simulink model "AGC30_PVcut_2021"  (R2021a)
settings: Solver=ode4  StartTime=stime  StopTime=etime  FixedStep=dtload  RelTol=1e-3
values from neighbouring files (symbols this model uses):
  AL_A = 0.3    [initset_lfc.m]
  AL_B = 0.3    [initset_lfc.m]
  DELTA_B = 0.067    [initset_otherarea.m]
  dtload = 0.1    [initset_dataload.m]
  F0 = 60    [initset_inertia.m]
  FFCS0_CC = (WF0_CC-WF_MIN_CC)./(1.0-WF_MIN_CC)    [init_thermals.m]
  FX_FB_ST_OA = Fx_fb_st_ty(:,TY_ST)    [initset_otherarea.m]
  FX_FB_WT = FX_FB_WT_ty(:,TY_WT)    [read_const_conhydros.m]
  FX_PTHD_ST_OA = Fx_pthd_st_ty(:,TY_ST)    [initset_otherarea.m]
  FY_FB_ST_OA = [1;1;0;0;-1;-1]*PLM_B    [initset_otherarea.m]
  FY_FB_WT = FY_FB_WT_ty(:,TY_WT)    [read_const_conhydros.m]
  FY_PTHD_ST_OA = [1;1;1;1]    [initset_otherarea.m]
  G_cost = [Cost(:,3) ... (first row only)    [initset_dataload.m]
  G_down_limit = max(G_down_limit, G_out_pre - G_speed*5)    [edc.m]    (also in initset_dataload.m = csvread('G_down_plan_limit.csv',0,1))
  G_G_ST_OA = G_g_st_ty(TY_ST)    [initset_otherarea.m]
  G_speed = u(220:249,1)    [edc.m]    (also in initset_dataload.m = G_speed(:,1))
  GF_CC = [1, 1, 1, 1, 1,            1, 1, 1, 1, 1]    [initset_thermals.m]
  GF_ST = [1, 1, 1, 1, 1, 1, 1,            1, 1, 1, 1,            1, 1, 1, 1, 1, 1]    [initset_thermals.m]
  GMW_WT = GMW_WT_ty(TY_WT)    [read_const_conhydros.m]
  IGV0_CC = WF0_CC    [init_thermals.m]
  inertia_input = [1 31.872 31.872 2 31.872 31.872 3 31.872 31.872 4 31.872 31.872 ... (259203 elements, 3x86401)]    [inertia_input.mat]    (also in initset_dataload.m = inertia_input')
  K1_CONV_WT = K1_CONV_WT_ty(TY_WT)    [read_const_conhydros.m]
  K2_SERV_WT = K2_SERV_WT_ty(TY_WT)    [read_const_conhydros.m]
  K_A = 0.1    [initset_lfc.m]
  K_B = 0.1    [initset_lfc.m]
  K_G_ST_OA = K_g_st_ty(TY_ST)    [initset_otherarea.m]
  K_L = 2.0    (= 2)    [initset_inertia.m]
  K_PREF_ST_OA = K_pref_st_ty(TY_ST)    [initset_otherarea.m]
  K_SD_WT = K_SD_WT_ty(TY_WT)    [read_const_conhydros.m]
  K_SEQ_WT = K_SEQ_WT_ty(TY_WT)    [read_const_conhydros.m]
  KD_PID_WT = KD_PID_WT_ty(TY_WT)    [read_const_conhydros.m]
  KGT_CC = FGT_CC./((TFR_CC-TER_CC)-(TDR_CC-TIR_CC))    [init_thermals.m]
  KI_PID_WT = KI_PID_WT_ty(TY_WT)    [read_const_conhydros.m]
  KP_A = 1.0    (= 1)    [initset_lfc.m]
  KP_B = 1.0    (= 1)    [initset_lfc.m]
  KP_PID_WT = KP_PID_WT_ty(TY_WT)    [read_const_conhydros.m]
  KST_CC = (1.0-FGT_CC)./TER_CC    [init_thermals.m]
  L_MWD_WT = L_MWD_WT_ty(TY_WT)    [read_const_conhydros.m]
  LFC_cycle = 5.0    (= 5)    [initset_lfc.m]
  load_input = load_input(:,stime+1:etime+1)    [initset_dataload.m]
  MVABase = 1000    [initset_inertia.m]
  MW0_ST = zeros(1,17)    [init_thermals.m]
  MW0_WT = zeros(1,2)    [init_conhydros.m]
  P_G_CONV_WT = P_G_CONV_WT_ty(TY_WT)    [read_const_conhydros.m]
  PG_INIT_CC = PMWD_SCHEDULE(1,19:28)'    [init_thermals.m]
  PLM_B = 0.03    [initset_otherarea.m]
  PMAX_B = 360.0    (= 360)    [initset_lfc.m]
  PMIN_B = -360.0    (= -360)    [initset_lfc.m]
  PMST0_CC = zeros(1, 10)    [init_thermals.m]
  PMWD_EDC0 = zeros(1,30)    [initset_edc.m]
  PMWD_SCHEDULE = u(3:32,1)    [edc.m]    (also in initset_edc.m = g_out_input')
  PRT_CC = PRC_CC.*(1-EP_CC)    [init_thermals.m]
  PTH0_ST = zeros(1,17)    [init_thermals.m]
  R_LL_ST_OA = R_ll_st_ty(TY_ST)    [initset_otherarea.m]
  RA_A = G_speed'    [initset_lfc.m]
  RA_B = 96.0    (= 96)    [initset_lfc.m]
  T1_B_ST_OA = T1_b_st_ty(TY_ST)    [initset_otherarea.m]
  T1_CONV_WT = T1_CONV_WT_ty(TY_WT)    [read_const_conhydros.m]
  T1_G_ST_OA = T1_g_st_ty(TY_ST)    [initset_otherarea.m]
  T2_B_ST_OA = T2_b_st_ty(TY_ST)    [initset_otherarea.m]
  T2_G_ST_OA = T2_g_st_ty(TY_ST)    [initset_otherarea.m]
  T2_SERV_WT = T2_SERV_WT_ty(TY_WT)    [read_const_conhydros.m]
  T3_B_ST_OA = T3_b_st_ty(TY_ST)    [initset_otherarea.m]
  T3_SERV_WT = T3_SERV_WT_ty(TY_WT)    [read_const_conhydros.m]
  T4_G_ST_OA = T4_g_st_ty(TY_ST)    [initset_otherarea.m]
  T5_G_ST_OA = T5_g_st_ty(TY_ST)    [initset_otherarea.m]
  T_0 = 2.5    [initset_trfpP.m]
  T_LL_ST_OA = T_ll_st_ty(TY_ST)    [initset_otherarea.m]
  T_PREF_ST_OA = T_pref_st_ty(TY_ST)    [initset_otherarea.m]
  TD_PID_WT = TD_PID_WT_ty(TY_WT)    [read_const_conhydros.m]
  TDR_CC = TIR_CC.*(1+(PRC_CC.^((RC_CC-1)./RC_CC)-1)./HC_CC)    [init_thermals.m]
  TE0_CC = zeros(1, 10)    [init_thermals.m]
  TER_CC = TFR_CC.*(1-(1-1./PRT_CC.^((RT_CC-1)./RT_CC)).*HT_CC)    [init_thermals.m]
  Tieline_Base = [1 0 2 0 3 0 4 0 5 0 6 0 ... (172802 elements, 2x86401)]    [Tieline_Base.mat]    (also in initset_dataload.m = Tieline_Base')
  TW_WAY_WT = TW_WAY_WT_ty(TY_WT)    [read_const_conhydros.m]
  U_MWD_WT = U_MWD_WT_ty(TY_WT)    [read_const_conhydros.m]
  WF0_CC = 1.0*ones(1, 10)    [init_thermals.m]
  WF_MIN_CC = L_IGV_CC./(TFR_CC-TDR_CC).*((Td_min_cc-TIR_CC)     ./((1-1./(PRT_CC.*L_IGV_CC).^((RT_CC-1)./RT_CC)).*HT_CC)-Td_min_cc)    [init_thermals.m]
  XAR_A = 10.0    (= 10)    [initset_lfc.m]
  XAR_B = 10.0    (= 10)    [initset_lfc.m]
  XF_A = 0.00    (= 0)    [initset_lfc.m]
  XF_B = 0.00    (= 0)    [initset_lfc.m]
undefined symbols (not defined in the file or in its folder): DELTA_CC, DELTA_ST, DiscIntNeverNeededParam, FGT_CC, FX_FB_CC, FX_FB_ST, FX_N_GN_VA, FX_N_PM_VA, FX_PTHD_ST, FX_T_PM_VA, FX_TE1_CC, FX_TE2_CC, FX_Y_GN_VA, FX_Y_PM_VA, FY_FB_CC, FY_FB_ST, FY_N_GN_VA, FY_N_PM_VA, FY_PTHD_ST, FY_T_PM_VA, FY_TE1_CC, FY_TE2_CC, FY_Y_GN_VA, FY_Y_PM_VA, G_G_ST, GMW_CC, GMW_ST, GMW_VA, HC_CC, HT_CC, K1_CONV_VA, K2_SERV_VA, K_G_ST, K_IGV_CC, K_MW_GV_VA, K_PREF_ST, K_SD_VA, K_TE_CC, KD_PID_VA, KD_SG_GN_VA, KD_SG_PM_VA, KI_PID_VA, KI_SG_GN_VA, KI_SG_PM_VA, KP_PID_VA, KP_SG_GN_VA, KP_SG_PM_VA, L_FUEL_CC, L_G_ST, L_IGV_CC, L_LL_ST, L_MWD_CC, L_MWD_GN_VA, L_MWD_PM_VA, L_MWD_ST, L_PREF_CC, L_PREF_ST, M_VA, MW0_ST_OA, N_GN_INIT_VA ... (+56)
libraries: simulink_extras x87, simulink x43, eeGeneralControl x2, pid_lib x1
(part 2 of 4)

== system AGC30_PVcut_2021/他エリア発電プラント/他エリアモデル ==
  EDC指令値(MW) : Inport
  LFC指令値(MW) : Inport  Port=2
  周波数偏差(Hz) : Inport  Port=3
  Add2 : Sum
  Add3 : Sum
  CVサーボ時定数 : Gain  Gain=1/T2_G_ST_OA(1)
  GF・LL幅 : Constant  Value=PLM_B
  Hz->pu : Gain  Gain=1/F0
  MW->pu : Product  Inputs=/*
  MWD' : Sum
  MWD(MW) : Sum
  MinMax : MinMax  Inputs=2
  Mux1 : Mux  Inputs=3
  Scope : Scope
  Subtract : Sum  Inputs=+-
  Subtract1 : Sum  Inputs=+-
  Subtract2 : Sum  Inputs=+-
  pu->MW : Product  RndMeth=Zero
  スピードリレー : TransferFcn  Numerator=[G_G_ST_OA(1) 1]  Denominator=[T1_G_ST_OA(1) 1]
  タービン出力 : Sum
  ボイラ特性 : simulink_extras/Additional Linear/Transfer Fcn (with initial outputs)  N=[1]  D=[T2_B_ST_OA(1) 1]  Y0=0  U0=0
  ボイラ発生蒸気 : simulink_extras/Additional Linear/Transfer Fcn (with initial outputs)  N=[1]  D=[T1_B_ST_OA(1) 1]  Y0=MW0_ST_OA(1)  U0=MW0_ST_OA(1)
  中低圧タービン・再熱器 : simulink_extras/Additional Linear/Transfer Fcn (with initial outputs)  N=[1]  D=[T5_G_ST_OA(1) 1]  Y0=MW0_ST_OA(1)  U0=MW0_ST_OA(1)
  中低圧タービン分担比 : Gain  Gain=1.0-K_G_ST_OA(1)
  主蒸気圧力 : Sum
  主蒸気圧力 偏差 : Sum  Inputs=+-
  主蒸気圧力設定 : Lookup  InputValues=FX_PTHD_ST_OA(:,1)  Table=FY_PTHD_ST_OA(:,1)  LookUpMeth=Interpolation-Use End Values
  主蒸気流量 : Product  RndMeth=Zero
  他エリア出力 : ToWorkspace  VariableName=OtherArea_Out  SampleTime=-1
      settings: Save2DSignal=2-D array (concatenate along first dimension)
  出力偏差 : Sum  Inputs=-++
  出力制御積分 : Integrator  InitialCondition=1.0  UpperSaturationLimit=Inf  LowerSaturationLimit=0
  周波数バイアス : Lookup  InputValues=FX_FB_ST_OA(:,1)/F0  Table=FY_FB_ST_OA(:,1)  LookUpMeth=Interpolation-Use End Values
  圧力制御 : simulink_extras/Additional Linear/Transfer Fcn (with initial outputs)  N=[1]  D=[T3_B_ST_OA(1) 1]  Y0=0  U0=0
  比例ゲイン : Gain  Gain=K_PREF_ST_OA(1)
  積分時定数 : Gain  Gain=1/T_PREF_ST_OA(1)
  蒸気加減弁開度 : Integrator  InitialCondition=1.0  UpperSaturationLimit=Inf  LowerSaturationLimit=0
  追従回路 : Subsystem
  速度調定率 : Gain  Gain=1.0/DELTA_B
  高圧タービン : simulink_extras/Additional Linear/Transfer Fcn (with initial outputs)  N=[1]  D=[T4_G_ST_OA(1) 1]  Y0=MW0_ST_OA(1)  U0=MW0_ST_OA(1)
  高圧タービン分担比 : Gain  Gain=K_G_ST_OA(1)
  タービン出力(MW) : Outport  VectorParamsAs1DForOutWhenUnconnected=off
  wires:
  MWD(MW)/1 -> MW->pu/2
  周波数偏差(Hz)/1 -> Hz->pu/1
  MWD'/1 -> ボイラ発生蒸気/1, 出力偏差/2
  ボイラ発生蒸気/1 -> Subtract/1, 主蒸気圧力設定/1
  出力偏差/1 -> 比例ゲイン/1, 積分時定数/1
  比例ゲイン/1 -> Add3/1
  主蒸気圧力 偏差/1 -> 主蒸気圧力/1, 出力偏差/3
  主蒸気圧力設定/1 -> 主蒸気圧力/2
  主蒸気流量/1 -> Subtract/2, 高圧タービン/1
  積分時定数/1 -> 出力制御積分/1
  出力制御積分/1 -> Add3/2
  速度調定率/1 -> スピードリレー/1
  Subtract1/1 -> MinMax/2
  主蒸気圧力/1 -> 主蒸気流量/1
  スピードリレー/1 -> Subtract1/2
  MinMax/1 -> Subtract2/1, Add2/2
  Subtract2/1 -> CVサーボ時定数/1
  CVサーボ時定数/1 -> 蒸気加減弁開度/1
  蒸気加減弁開度/1 -> 主蒸気流量/2, Subtract2/2
  高圧タービン/1 -> 中低圧タービン・再熱器/1, 高圧タービン分担比/1
  中低圧タービン・再熱器/1 -> 中低圧タービン分担比/1
  高圧タービン分担比/1 -> タービン出力/2
  中低圧タービン分担比/1 -> タービン出力/1
  タービン出力/1 -> pu->MW/1, 出力偏差/1
  GF・LL幅/1 -> Add2/1
  Add2/1 -> 追従回路/1(In)
  ボイラ特性/1 -> 主蒸気圧力 偏差/1
  圧力制御/1 -> 主蒸気圧力 偏差/2
  Subtract/1 -> ボイラ特性/1, 圧力制御/1
  Add3/1 -> Subtract1/1
  Hz->pu/1 -> 速度調定率/1, 周波数バイアス/1
  EDC指令値(MW)/1 -> Mux1/1, MW->pu/1, MWD(MW)/1, pu->MW/2
  LFC指令値(MW)/1 -> Mux1/2, MWD(MW)/2
  追従回路/1(Out) -> MinMax/1
  周波数バイアス/1 -> MWD'/1
  Mux1/1 -> 他エリア出力/1
  MW->pu/1 -> MWD'/2
  pu->MW/1 -> Scope/1, Mux1/3, タービン出力(MW)/1

== system AGC30_PVcut_2021/可変速揚水発電機/可変速揚水 ==
  note: EDCとLFC指令の入力方法を変更
  EDC指令値 (MW) : Inport
  LFC指令値 (MW) : Inport  Port=2
  周波数偏差 (Hz) : Inport  Port=3
  "  ±1  " : Saturate  UpperLimit=1  LowerLimit=-1
  " ±1 " : Integrator  LimitOutput=on  UpperSaturationLimit=1  LowerSaturationLimit=-1
  Abs : Abs
  Constant : Constant  Value=0
  EDC_Wt3 : Selector  InputPortWidth=AGCNum_E  IndexOptions=Index vector (dialog)  Indices=[30]  OutputSizes=1
  "Hz -> PU" : Gain  Gain=1/F0
  If : If  IfExpression=u1 >= 0
  LFC_Wt3 : Selector  InputPortWidth=AGCNum_L  IndexOptions=Index vector (dialog)  Indices=[30]  OutputSizes=1
  "MW -> PU" : Gain  Gain=1/GMW_VA(1)
  "PU -> MW" : Gain  Gain=GMW_VA(1)
  "SW " : Switch  Criteria=u2 > Threshold
  Scope{,1,3..6} (6 alike) : Scope
  Sum : Sum  Inputs=+++
  Sum2 : Sum  Inputs=|+-
  Sum3 : Sum  Inputs=|+-
  Sum4 : Sum
  Sum6 : Sum  Inputs=+|+
  ±1 : Saturate  UpperLimit=1  LowerLimit=-1
  微分 （リセットフィルタ） : TransferFcn  Numerator="[TD_PID_VA(1)  0]"  Denominator="[TD_PID_VA(1)  1]"
  微分ゲイン : Gain  Gain=KD_PID_VA(1)
  揚水運転 : Subsystem  TreatAsAtomicUnit=on
  比例ゲイン : Gain  Gain=KP_PID_VA(1)
  発電運転 : Subsystem  TreatAsAtomicUnit=on
  積分ゲイン : Gain  Gain=KI_PID_VA(1)
  速度調停率 : Gain  Gain=K_SD_VA(1)
  連続出力切替 : Subsystem
  運転モード : simulink/Logic and Bit Operations/Compare To Constant  relop=>=  const=GMW_VA(1)*L_MWD_GN_VA(1)  OutDataTypeStr=boolean
  発電機出力・揚水入力 (MW) : Outport  VectorParamsAs1DForOutWhenUnconnected=off
  wires:
  "MW -> PU"/1 -> Scope4/1, Sum2/1, 連続出力切替/3(MWD)
  EDC_Wt3/1 -> Abs/1, Scope6/1, 運転モード/1, Sum4/1
  Sum4/1 -> "MW -> PU"/1
  比例ゲイン/1 -> ±1/1
  Sum3/1 -> 微分ゲイン/1, 積分ゲイン/1, 比例ゲイン/1
  ±1/1 -> Sum/1
  " ±1 "/1 -> Sum/2
  積分ゲイン/1 -> " ±1 "/1
  EDC指令値 (MW)/1 -> EDC_Wt3/1
  "PU -> MW"/1 -> 発電機出力・揚水入力 (MW)/1
  連続出力切替/1(出力) -> "PU -> MW"/1
  揚水運転/1(Out2) -> Sum6/2, Scope1/1
  Sum6/1 -> Scope3/1, 連続出力切替/1(モデル)
  LFC_Wt3/1 -> Sum4/2
  LFC指令値 (MW)/1 -> LFC_Wt3/1
  微分ゲイン/1 -> 微分 （リセットフィルタ）/1
  運転モード/1 -> Scope5/1, 連続出力切替/2(運転モード)
  "  ±1  "/1 -> Sum/3
  速度調停率/1 -> Sum3/2
  "Hz -> PU"/1 -> Sum3/1
  周波数偏差 (Hz)/1 -> "Hz -> PU"/1
  微分 （リセットフィルタ）/1 -> "  ±1  "/1
  Sum/1 -> Sum2/2, 速度調停率/1
  Sum2/1 -> "SW "/1  "有効電力指令"
  Constant/1 -> "SW "/3
  Abs/1 -> "SW "/2
  If/1 -> 発電運転/Action
  If/2 -> 揚水運転/Action
  "SW "/1 -> 発電運転/1(In1), 揚水運転/1(In1), If/1
  発電運転/1(Out1) -> Scope/1, Sum6/1

== system AGC30_PVcut_2021/定速揚水発電プラント/Water1 ==
  note: IMAICHI P/S DYNAMIC BLOCK (imaichtd)
  EDC指令値(MW) : Inport
  LFC指令値(MW)1 : Inport  Port=2
  周波数偏差(Hz)1 : Inport  Port=3
  (1-TWs)/(1+0.5TWs) : simulink_extras/Additional Linear/Transfer Fcn (with initial outputs)  N=[-TW_WAY_WT(1) 1]  D=[TW_WAY_WT(1)/2 1]  Y0=MW0_WT(1)  U0=MW0_WT(1)
  Add : Sum
  Hz->pu : Gain  Gain=1/F0
  K1/(1+T1s)1 : simulink_extras/Additional Linear/Transfer Fcn (with initial outputs)  N=[K1_CONV_WT(1)]  D=[T1_CONV_WT(1) 1]  Y0=MW0_WT(1)/P_G_CONV_WT(1)  U0=MW0_WT(1)/P_G_CONV_WT(1)
  K2/(1+T2s+T3s^2)1 : simulink_extras/Additional Linear/Transfer Fcn (with initial outputs)  N=[K2_SERV_WT(1)]  D=[T3_SERV_WT(1) T2_SERV_WT(1) 1]  Y0=MW0_WT(1)/P_G_CONV_WT(1)  U0=MW0_WT(1)/P_G_CONV_WT(1)
  Kc/Tc (1/90) : Gain  Gain=K_SEQ_WT(1)  SaturateOnIntegerOverflow=on  OutDataTypeStr=Inherit: Same as input  ParamDataTypeStr=Inherit: Same as input
  Kd : Gain  Gain=KD_PID_WT(1)  SaturateOnIntegerOverflow=on  OutDataTypeStr=Inherit: Same as input  ParamDataTypeStr=Inherit: Same as input
  Ki : Gain  Gain=KI_PID_WT(1)  SaturateOnIntegerOverflow=on  OutDataTypeStr=Inherit: Same as input  ParamDataTypeStr=Inherit: Same as input
  Kp : Gain  Gain=KP_PID_WT(1)  SaturateOnIntegerOverflow=on  OutDataTypeStr=Inherit: Same as input  ParamDataTypeStr=Inherit: Same as input
  Ksd : Gain  Gain=K_SD_WT(1)  SaturateOnIntegerOverflow=on  OutDataTypeStr=Inherit: Same as input  ParamDataTypeStr=Inherit: Same as input
  MW->pu : Gain  Gain=1/GMW_WT(1)
  MWD(MW) : Sum
  Scope : Scope
  Scope1 : Scope
  Scope2 : Scope
  Scope4 : Scope  Commented=on
  Scope5 : Scope  Commented=on
  Sum12 : Sum  Inputs=-+  InputSameDT=on  SaturateOnIntegerOverflow=on  OutDataTypeStr=Inherit: Same as first input
  Sum17 : Sum  Inputs=-+  InputSameDT=on  SaturateOnIntegerOverflow=on  OutDataTypeStr=Inherit: Same as first input
  Sum18 : Sum  Inputs=-+  InputSameDT=on  SaturateOnIntegerOverflow=on  OutDataTypeStr=Inherit: Same as first input
  Sum19 : Sum  Inputs=+++  InputSameDT=on  SaturateOnIntegerOverflow=on  OutDataTypeStr=Inherit: Same as first input
  Tds/(1+Tds) : TransferFcn  Numerator=[TD_PID_WT(1) 0]  Denominator=[TD_PID_WT(1) 1]
  To Workspace : ToWorkspace  Commented=on  VariableName=PG1  SampleTime=-1
  To Workspace1 : ToWorkspace  Commented=on  VariableName=ELD  SampleTime=-1
  U=1  L=0 : Saturate  UpperLimit=1.  LowerLimit=0
  U=1 L=0 : Saturate  UpperLimit=1.  LowerLimit=0
  U=1.2L=1 : Subsystem  mask(Limited Integrator.){lower_limit=0, upper_limit=1.2, X0=MW0_WT(1)/P_G_CONV_WT(1)}
      mask prompts: lower_limit "Lower bound:"; upper_limit "Upper bound:"; X0 "Initial condition:"
      mask help: Limited Integrator
      mask Help: Implements a limited integrator with \nan expression of the form:\n\nif(x<=lb and u<0) or (x>=ub and u>0)\n   xdot=0\nelse\n   xdot=u
      mask Display: plot(-1,-0.2,3.5,1.2,[0.05,1,2,2.9],[0,0,1,1]);disp(' 1/s    ')
  U=1L=0 : Subsystem  mask(Limited Integrator.){lower_limit=0, upper_limit=1., X0=MW0_WT(1)/P_G_CONV_WT(1)}
      mask prompts: lower_limit "Lower bound:"; upper_limit "Upper bound:"; X0 "Initial condition:"
      mask help: Limited Integrator
      mask Help: Implements a limited integrator with \nan expression of the form:\n\nif(x<=lb and u<0) or (x>=ub and u>0)\n   xdot=0\nelse\n   xdot=u
      mask Display: plot(-1,-0.2,3.5,1.2,[0.05,1,2,2.9],[0,0,1,1]);disp(' 1/s    ')
  pu->MW : Gain  Gain=GMW_WT(1)  SaturateOnIntegerOverflow=on  OutDataTypeStr=Inherit: Same as input  ParamDataTypeStr=Inherit: Same as input
  puMW/puGV : Gain  Gain=P_G_CONV_WT(1)  SaturateOnIntegerOverflow=on  OutDataTypeStr=Inherit: Same as input  ParamDataTypeStr=Inherit: Same as input
  ±0.05 : Saturate  UpperLimit=0.05  LowerLimit=-0.05
  ±1 : Saturate  UpperLimit=1.  LowerLimit=-1.
  "±1 " : Saturate  UpperLimit=1.  LowerLimit=-1.
  出力上下限 : Saturate  UpperLimit=U_MWD_WT(1)  LowerLimit=L_MWD_WT(1)
  周波数バイアス : Lookup  InputValues=FX_FB_WT(:,1)/F0  Table=FY_FB_WT(:,1)  LookUpMeth=Interpolation-Use End Values
  連続出力切替 : Subsystem
  運転モード : simulink/Logic and Bit Operations/Compare To Constant  relop=>=  const=L_MWD_WT(1)*GMW_WT(1)  OutDataTypeStr=boolean
  タービン出力(MW) : Outport  VectorParamsAs1DForOutWhenUnconnected=off
  wires:
  ±0.05/1 -> Kc/Tc (1/90)/1
  Kc/Tc (1/90)/1 -> U=1.2L=1/1(Inport)
  U=1 L=0/1 -> Sum17/1, K2/(1+T2s+T3s^2)1/1
  Sum19/1 -> K1/(1+T1s)1/1
  U=1L=0/1(Outport) -> Sum19/2
  ±1/1 -> Sum19/1
  "±1 "/1 -> Sum19/3
  Tds/(1+Tds)/1 -> "±1 "/1
  Kd/1 -> Tds/(1+Tds)/1
  Kp/1 -> ±1/1
  Ki/1 -> U=1L=0/1(Inport)
  Sum17/1 -> Ksd/1
  Sum12/1 -> ±0.05/1
  Sum18/1 -> Ki/1, Kd/1, Kp/1
  U=1.2L=1/1(Outport) -> Sum17/2
  Ksd/1 -> Sum18/2
  K1/(1+T1s)1/1 -> U=1 L=0/1
  K2/(1+T2s+T3s^2)1/1 -> U=1  L=0/1
  出力上下限/1 -> Sum12/2
  EDC指令値(MW)/1 -> MWD(MW)/1, 運転モード/1, Scope2/1, To Workspace1/1
  LFC指令値(MW)1/1 -> MWD(MW)/2
  MWD(MW)/1 -> MW->pu/1
  周波数偏差(Hz)1/1 -> Hz->pu/1
  Hz->pu/1 -> 周波数バイアス/1, Sum18/1, Scope/1
  周波数バイアス/1 -> Add/2, Scope4/1
  MW->pu/1 -> Add/1, Scope1/1, 連続出力切替/3(MWD)
  Add/1 -> 出力上下限/1, Scope5/1
  U=1  L=0/1 -> puMW/puGV/1
  puMW/puGV/1 -> (1-TWs)/(1+0.5TWs)/1
  (1-TWs)/(1+0.5TWs)/1 -> Sum12/1, 連続出力切替/1(モデル)
  運転モード/1 -> 連続出力切替/2(運転モード)
  pu->MW/1 -> タービン出力(MW)/1, To Workspace/1
  連続出力切替/1(出力) -> pu->MW/1

== system AGC30_PVcut_2021/定速揚水発電プラント/Water2 ==
  EDC指令値(MW) : Inport
  LFC指令値(MW)1 : Inport  Port=2
  周波数偏差(Hz)1 : Inport  Port=3
  (1-TWs)/(1+0.5TWs) : simulink_extras/Additional Linear/Transfer Fcn (with initial outputs)  N=[-TW_WAY_WT(2) 1]  D=[TW_WAY_WT(2)/2 1]  Y0=MW0_WT(2)  U0=MW0_WT(2)
  Add : Sum
  Hz->pu : Gain  Gain=1/F0
  K1/(1+T1s)1 : simulink_extras/Additional Linear/Transfer Fcn (with initial outputs)  N=[K1_CONV_WT(2)]  D=[T1_CONV_WT(2) 1]  Y0=MW0_WT(2)/P_G_CONV_WT(2)  U0=MW0_WT(2)/P_G_CONV_WT(2)
  K2/(1+T2s+T3s^2)1 : simulink_extras/Additional Linear/Transfer Fcn (with initial outputs)  N=[K2_SERV_WT(2)]  D=[T3_SERV_WT(2) T2_SERV_WT(2) 1]  Y0=MW0_WT(2)/P_G_CONV_WT(2)  U0=MW0_WT(2)/P_G_CONV_WT(2)
  Kc/Tc (1/90) : Gain  Gain=K_SEQ_WT(2)  SaturateOnIntegerOverflow=on  OutDataTypeStr=Inherit: Same as input  ParamDataTypeStr=Inherit: Same as input
  Kd : Gain  Gain=KD_PID_WT(2)  SaturateOnIntegerOverflow=on  OutDataTypeStr=Inherit: Same as input  ParamDataTypeStr=Inherit: Same as input
  Ki : Gain  Gain=KI_PID_WT(2)  SaturateOnIntegerOverflow=on  OutDataTypeStr=Inherit: Same as input  ParamDataTypeStr=Inherit: Same as input
  Kp : Gain  Gain=KP_PID_WT(2)  SaturateOnIntegerOverflow=on  OutDataTypeStr=Inherit: Same as input  ParamDataTypeStr=Inherit: Same as input
  Ksd : Gain  Gain=K_SD_WT(2)  SaturateOnIntegerOverflow=on  OutDataTypeStr=Inherit: Same as input  ParamDataTypeStr=Inherit: Same as input
  MW->pu : Gain  Gain=1/GMW_WT(2)
  MWD(MW) : Sum
  Scope : Scope
  Scope1 : Scope  Commented=on
  Scope4 : Scope
  Scope5 : Scope  Commented=on
  Sum12 : Sum  Inputs=-+  InputSameDT=on  SaturateOnIntegerOverflow=on  OutDataTypeStr=Inherit: Same as first input
  Sum17 : Sum  Inputs=-+  InputSameDT=on  SaturateOnIntegerOverflow=on  OutDataTypeStr=Inherit: Same as first input
  Sum18 : Sum  Inputs=-+  InputSameDT=on  SaturateOnIntegerOverflow=on  OutDataTypeStr=Inherit: Same as first input
  Sum19 : Sum  Inputs=+++  InputSameDT=on  SaturateOnIntegerOverflow=on  OutDataTypeStr=Inherit: Same as first input
  Tds/(1+Tds) : TransferFcn  Numerator=[TD_PID_WT(2) 0]  Denominator=[TD_PID_WT(2) 1]
  U=1  L=0 : Saturate  UpperLimit=1.  LowerLimit=0
  U=1 L=0 : Saturate  UpperLimit=1.  LowerLimit=0
  U=1.2L=1 : Subsystem  mask(Limited Integrator.){lower_limit=0, upper_limit=1.2, X0=MW0_WT(2)/P_G_CONV_WT(2)}
      mask prompts: lower_limit "Lower bound:"; upper_limit "Upper bound:"; X0 "Initial condition:"
      mask help: Limited Integrator
      mask Help: Implements a limited integrator with \nan expression of the form:\n\nif(x<=lb and u<0) or (x>=ub and u>0)\n   xdot=0\nelse\n   xdot=u
      mask Display: plot(-1,-0.2,3.5,1.2,[0.05,1,2,2.9],[0,0,1,1]);disp(' 1/s    ')
  U=1L=0 : Subsystem  mask(Limited Integrator.){lower_limit=0, upper_limit=1., X0=MW0_WT(1)/P_G_CONV_WT(1)}
      mask prompts: lower_limit "Lower bound:"; upper_limit "Upper bound:"; X0 "Initial condition:"
      mask help: Limited Integrator
      mask Help: Implements a limited integrator with \nan expression of the form:\n\nif(x<=lb and u<0) or (x>=ub and u>0)\n   xdot=0\nelse\n   xdot=u
      mask Display: plot(-1,-0.2,3.5,1.2,[0.05,1,2,2.9],[0,0,1,1]);disp(' 1/s    ')
  pu->MW : Gain  Gain=GMW_WT(2)  SaturateOnIntegerOverflow=on  OutDataTypeStr=Inherit: Same as input  ParamDataTypeStr=Inherit: Same as input
  puMW/puGV : Gain  Gain=P_G_CONV_WT(2)  SaturateOnIntegerOverflow=on  OutDataTypeStr=Inherit: Same as input  ParamDataTypeStr=Inherit: Same as input
  ±0.05 : Saturate  UpperLimit=0.05  LowerLimit=-0.05
  ±1 : Saturate  UpperLimit=1.  LowerLimit=-1.
  "±1 " : Saturate  UpperLimit=1.  LowerLimit=-1.
  出力上下限 : Saturate  UpperLimit=U_MWD_WT(2)  LowerLimit=L_MWD_WT(2)
  周波数バイアス : Lookup  InputValues=FX_FB_WT(:,2)/F0  Table=FY_FB_WT(:,2)  LookUpMeth=Interpolation-Use End Values
  連続出力切替 : Subsystem
  運転モード : simulink/Logic and Bit Operations/Compare To Constant  relop=>=  const=L_MWD_WT(2)*GMW_WT(2)  OutDataTypeStr=boolean
  タービン出力(MW) : Outport  VectorParamsAs1DForOutWhenUnconnected=off
  wires:
  ±0.05/1 -> Kc/Tc (1/90)/1
  Kc/Tc (1/90)/1 -> U=1.2L=1/1(Inport)
  U=1 L=0/1 -> Sum17/1, K2/(1+T2s+T3s^2)1/1
  Sum19/1 -> K1/(1+T1s)1/1
  U=1L=0/1(Outport) -> Sum19/2
  ±1/1 -> Sum19/1
  "±1 "/1 -> Sum19/3
  Tds/(1+Tds)/1 -> "±1 "/1
  Kd/1 -> Tds/(1+Tds)/1
  Kp/1 -> ±1/1
  Ki/1 -> U=1L=0/1(Inport)
  Sum17/1 -> Ksd/1
  Sum12/1 -> ±0.05/1
  Sum18/1 -> Ki/1, Kd/1, Kp/1
  U=1.2L=1/1(Outport) -> Sum17/2
  Ksd/1 -> Sum18/2
  K1/(1+T1s)1/1 -> U=1 L=0/1
  K2/(1+T2s+T3s^2)1/1 -> U=1  L=0/1
  出力上下限/1 -> Sum12/2
  EDC指令値(MW)/1 -> MWD(MW)/1, 運転モード/1
  LFC指令値(MW)1/1 -> MWD(MW)/2
  MWD(MW)/1 -> MW->pu/1
  周波数偏差(Hz)1/1 -> Hz->pu/1
  Hz->pu/1 -> 周波数バイアス/1, Scope/1, Sum18/1
  周波数バイアス/1 -> Add/2, Scope4/1
  MW->pu/1 -> Add/1, Scope1/1, 連続出力切替/3(MWD)
  Add/1 -> 出力上下限/1, Scope5/1
  U=1  L=0/1 -> puMW/puGV/1
  puMW/puGV/1 -> (1-TWs)/(1+0.5TWs)/1
  (1-TWs)/(1+0.5TWs)/1 -> Sum12/1, 連続出力切替/1(モデル)
  運転モード/1 -> 連続出力切替/2(運転モード)
  連続出力切替/1(出力) -> pu->MW/1
  pu->MW/1 -> タービン出力(MW)/1

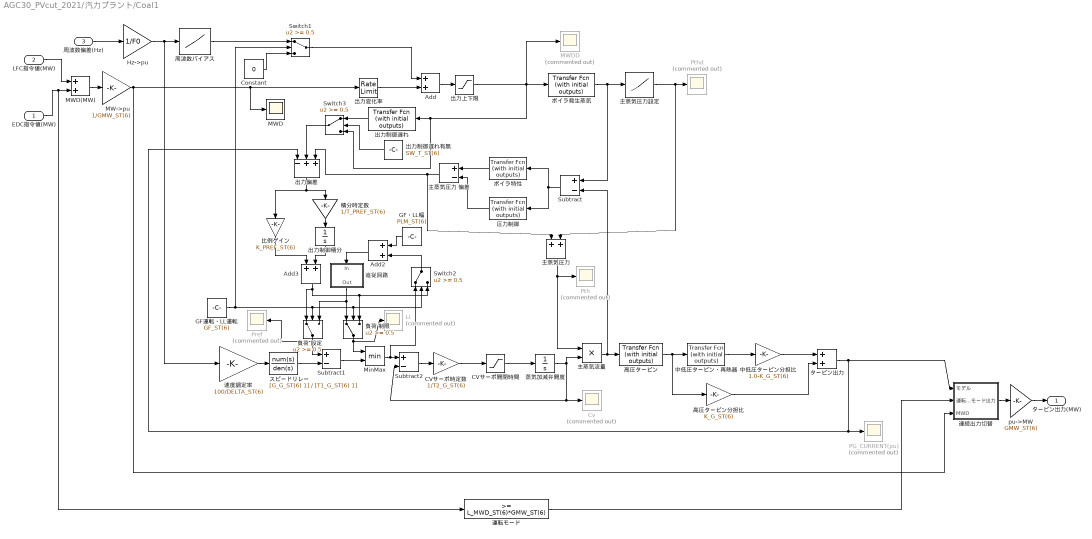
== system AGC30_PVcut_2021/汽力プラント/Coal1 ==
  EDC指令値(MW) : Inport
  LFC指令値(MW) : Inport  Port=2
  周波数偏差(Hz) : Inport  Port=3
  Add : Sum
  Add2 : Sum
  Add3 : Sum
  CVサーボ時定数 : Gain  Gain=1/T2_G_ST(6)
  CVサーボ開閉時間 : Saturate  UpperLimit=1/T3_G_ST(6)  LowerLimit=1/T6_G_ST(6)
  Constant : Constant  Value=0
  Cv : Scope  Commented=on
  GF・LL幅 : Constant  Value=PLM_ST(6)
  GF運転・LL運転 : Constant  Value=GF_ST(6)
  Hz->pu : Gain  Gain=1/F0
  Ll : Scope  Commented=on
  MW->pu : Gain  Gain=1/GMW_ST(6)
  MWD : Scope
  MWD(MW) : Sum
  MWDD : Scope  Commented=on
  MinMax : MinMax  Inputs=2
  PG_CURRENT(pu) : Scope  Commented=on
  Pref : Scope  Commented=on
  Pth : Scope  Commented=on
  Pthd : Scope  Commented=on
  Subtract : Sum  Inputs=+-
  Subtract1 : Sum  Inputs=+-
  Subtract2 : Sum  Inputs=+-
  Switch1 : Switch  Threshold=0.5
  Switch2 : Switch  Threshold=0.5
  Switch3 : Switch  Threshold=0.5
  pu->MW : Gain  Gain=GMW_ST(6)
  スピードリレー : TransferFcn  Numerator=[G_G_ST(6) 1]  Denominator=[T1_G_ST(6) 1]
  タービン出力 : Sum
  ボイラ特性 : simulink_extras/Additional Linear/Transfer Fcn (with initial outputs)  N=[1]  D=[T2_B_ST(6) 1]  Y0=0  U0=0
  ボイラ発生蒸気 : simulink_extras/Additional Linear/Transfer Fcn (with initial outputs)  N=[1]  D=[T1_B_ST(6) 1]  Y0=MW0_ST(6)  U0=MW0_ST(6)
  中低圧タービン・再熱器 : simulink_extras/Additional Linear/Transfer Fcn (with initial outputs)  N=[1]  D=[T5_G_ST(6) 1]  Y0=MW0_ST(6)  U0=MW0_ST(6)
  中低圧タービン分担比 : Gain  Gain=1.0-K_G_ST(6)
  主蒸気圧力 : Sum
  主蒸気圧力 偏差 : Sum  Inputs=+-
  主蒸気圧力設定 : Lookup  InputValues=FX_PTHD_ST(:,6)  Table=FY_PTHD_ST(:,6)  LookUpMeth=Interpolation-Use End Values
  主蒸気流量 : Product  RndMeth=Zero
  出力上下限 : Saturate  UpperLimit=U_MWD_ST(6)  LowerLimit=L_MWD_ST(6)
  出力偏差 : Sum  Inputs=-++
  出力制御積分 : Integrator  InitialCondition=MW0_ST(6)/PTH0_ST(6)  LimitOutput=on  UpperSaturationLimit=U_PREF_ST(6)  LowerSaturationLimit=L_PREF_ST(6)
  出力制御遅れ : simulink_extras/Additional Linear/Transfer Fcn (with initial outputs)  N=[1]  D=[T_T_ST(6) 1]  Y0=MW0_ST(6)  U0=MW0_ST(6)
  出力制御遅れ有無 : Constant  Value=SW_T_ST(6)
  出力変化率 : RateLimiter  RisingSlewLimit=R_MWD_ST(6)/60  FallingSlewLimit=-R_MWD_ST(6)/60  SampleTimeMode=inherited  InitialCondition=MW0_ST(6)
  周波数バイアス : Lookup  InputValues=FX_FB_ST(:,6)/F0  Table=FY_FB_ST(:,6)  LookUpMeth=Interpolation-Use End Values
  圧力制御 : simulink_extras/Additional Linear/Transfer Fcn (with initial outputs)  N=[1]  D=[T3_B_ST(6) 1]  Y0=0  U0=0
  比例ゲイン : Gain  Gain=K_PREF_ST(6)
  積分時定数 : Gain  Gain=1/T_PREF_ST(6)
  蒸気加減弁開度 : Integrator  InitialCondition=MW0_ST(6)/PTH0_ST(6)  LimitOutput=on  UpperSaturationLimit=U_G_ST(6)  LowerSaturationLimit=L_G_ST(6)
  負荷 制限 : Switch  Threshold=0.5
  負荷 設定 : Switch  Threshold=0.5
  追従回路 : Subsystem
  速度調定率 : Gain  Gain=100/DELTA_ST(6)
  連続出力切替 : Subsystem
  運転モード : simulink/Logic and Bit Operations/Compare To Constant  relop=>=  const=L_MWD_ST(6)*GMW_ST(6)  OutDataTypeStr=boolean
  高圧タービン : simulink_extras/Additional Linear/Transfer Fcn (with initial outputs)  N=[1]  D=[T4_G_ST(6) 1]  Y0=MW0_ST(6)  U0=MW0_ST(6)
  高圧タービン分担比 : Gain  Gain=K_G_ST(6)
  タービン出力(MW) : Outport  VectorParamsAs1DForOutWhenUnconnected=off
  wires:
  MWD(MW)/1 -> MW->pu/1
  周波数偏差(Hz)/1 -> Hz->pu/1
  Add/1 -> 出力上下限/1
  出力変化率/1 -> Add/2
  ボイラ発生蒸気/1 -> Subtract/1, 主蒸気圧力設定/1
  出力偏差/1 -> 比例ゲイン/1, 積分時定数/1
  比例ゲイン/1 -> Add3/1
  Add3/1 -> 負荷 制限/3, Switch2/3, 負荷 設定/1
  主蒸気圧力 偏差/1 -> 主蒸気圧力/1, 出力偏差/3
  主蒸気圧力設定/1 -> Pthd/1, 主蒸気圧力/2
  主蒸気流量/1 -> Subtract/2, 高圧タービン/1
  積分時定数/1 -> 出力制御積分/1
  出力制御積分/1 -> Add3/2
  速度調定率/1 -> スピードリレー/1
  Subtract1/1 -> MinMax/2
  主蒸気圧力/1 -> 主蒸気流量/1, Pth/1
  スピードリレー/1 -> Subtract1/2
  MinMax/1 -> Subtract2/1, Switch2/1
  Subtract2/1 -> CVサーボ時定数/1
  CVサーボ時定数/1 -> CVサーボ開閉時間/1
  CVサーボ開閉時間/1 -> 蒸気加減弁開度/1
  蒸気加減弁開度/1 -> 主蒸気流量/2, Subtract2/2, Cv/1
  高圧タービン/1 -> 中低圧タービン・再熱器/1, 高圧タービン分担比/1
  中低圧タービン・再熱器/1 -> 中低圧タービン分担比/1
  高圧タービン分担比/1 -> タービン出力/2
  中低圧タービン分担比/1 -> タービン出力/1
  タービン出力/1 -> 出力偏差/1, PG_CURRENT(pu)/1, 連続出力切替/1(モデル)
  GF・LL幅/1 -> Add2/1
  Add2/1 -> 追従回路/1(In)
  ボイラ特性/1 -> 主蒸気圧力 偏差/1
  圧力制御/1 -> 主蒸気圧力 偏差/2
  Subtract/1 -> ボイラ特性/1, 圧力制御/1
  出力上下限/1 -> ボイラ発生蒸気/1, MWDD/1, 出力制御遅れ/1, Switch3/3
  GF運転・LL運転/1 -> 負荷 設定/2, 負荷 制限/2, Switch2/2, Switch1/2
  負荷 設定/1 -> Subtract1/1, Pref/1
  追従回路/1(Out) -> 負荷 制限/1, 負荷 設定/3
  Switch2/1 -> Add2/2
  MW->pu/1 -> MWD/1, 出力変化率/1, 連続出力切替/3(MWD)
  Hz->pu/1 -> 速度調定率/1, 周波数バイアス/1
  連続出力切替/1(出力) -> pu->MW/1
  pu->MW/1 -> タービン出力(MW)/1
  負荷 制限/1 -> MinMax/1, Ll/1
  周波数バイアス/1 -> Switch1/1
  Constant/1 -> Switch1/3
  Switch1/1 -> Add/1
  出力制御遅れ/1 -> Switch3/1
  Switch3/1 -> 出力偏差/2
  出力制御遅れ有無/1 -> Switch3/2
  EDC指令値(MW)/1 -> MWD(MW)/2, 運転モード/1
  LFC指令値(MW)/1 -> MWD(MW)/1
  運転モード/1 -> 連続出力切替/2(運転モード)

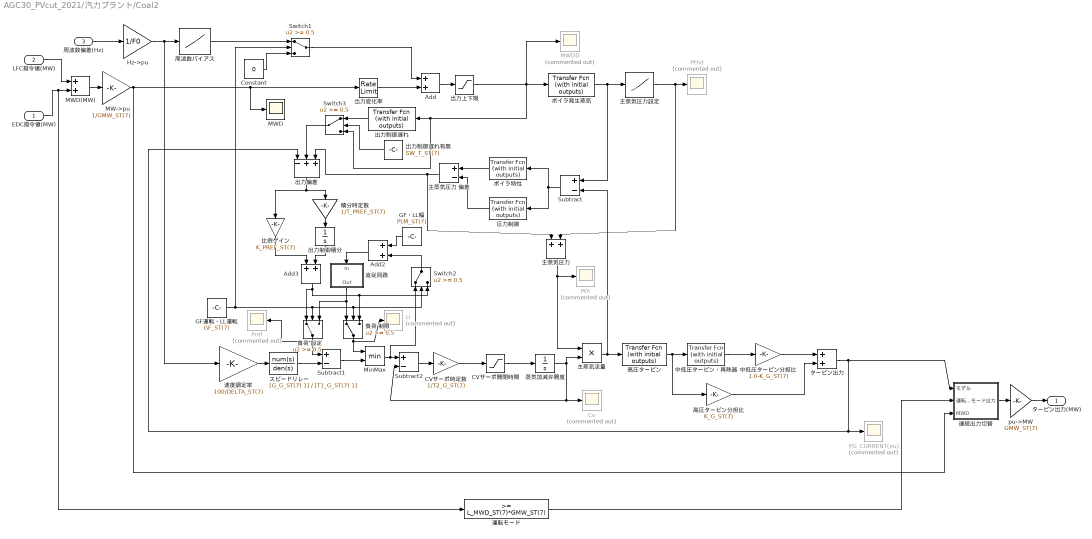
== system AGC30_PVcut_2021/汽力プラント/Coal2 ==
  EDC指令値(MW) : Inport
  LFC指令値(MW) : Inport  Port=2
  周波数偏差(Hz) : Inport  Port=3
  Add : Sum
  Add2 : Sum
  Add3 : Sum
  CVサーボ時定数 : Gain  Gain=1/T2_G_ST(7)
  CVサーボ開閉時間 : Saturate  UpperLimit=1/T3_G_ST(7)  LowerLimit=1/T6_G_ST(7)
  Constant : Constant  Value=0
  Cv : Scope  Commented=on
  GF・LL幅 : Constant  Value=PLM_ST(7)
  GF運転・LL運転 : Constant  Value=GF_ST(7)
  Hz->pu : Gain  Gain=1/F0
  Ll : Scope  Commented=on
  MW->pu : Gain  Gain=1/GMW_ST(7)
  MWD : Scope
  MWD(MW) : Sum
  MWDD : Scope  Commented=on
  MinMax : MinMax  Inputs=2
  PG_CURRENT(pu) : Scope  Commented=on
  Pref : Scope  Commented=on
  Pth : Scope  Commented=on
  Pthd : Scope  Commented=on
  Subtract : Sum  Inputs=+-
  Subtract1 : Sum  Inputs=+-
  Subtract2 : Sum  Inputs=+-
  Switch1 : Switch  Threshold=0.5
  Switch2 : Switch  Threshold=0.5
  Switch3 : Switch  Threshold=0.5
  pu->MW : Gain  Gain=GMW_ST(7)
  スピードリレー : TransferFcn  Numerator=[G_G_ST(7) 1]  Denominator=[T1_G_ST(7) 1]
  タービン出力 : Sum
  ボイラ特性 : simulink_extras/Additional Linear/Transfer Fcn (with initial outputs)  N=[1]  D=[T2_B_ST(7) 1]  Y0=0  U0=0
  ボイラ発生蒸気 : simulink_extras/Additional Linear/Transfer Fcn (with initial outputs)  N=[1]  D=[T1_B_ST(7) 1]  Y0=MW0_ST(7)  U0=MW0_ST(7)
  中低圧タービン・再熱器 : simulink_extras/Additional Linear/Transfer Fcn (with initial outputs)  N=[1]  D=[T5_G_ST(7) 1]  Y0=MW0_ST(7)  U0=MW0_ST(7)
  中低圧タービン分担比 : Gain  Gain=1.0-K_G_ST(7)
  主蒸気圧力 : Sum
  主蒸気圧力 偏差 : Sum  Inputs=+-
  主蒸気圧力設定 : Lookup  InputValues=FX_PTHD_ST(:,7)  Table=FY_PTHD_ST(:,7)  LookUpMeth=Interpolation-Use End Values
  主蒸気流量 : Product  RndMeth=Zero
  出力上下限 : Saturate  UpperLimit=U_MWD_ST(7)  LowerLimit=L_MWD_ST(7)
  出力偏差 : Sum  Inputs=-++
  出力制御積分 : Integrator  InitialCondition=MW0_ST(7)/PTH0_ST(7)  LimitOutput=on  UpperSaturationLimit=U_PREF_ST(7)  LowerSaturationLimit=L_PREF_ST(7)
  出力制御遅れ : simulink_extras/Additional Linear/Transfer Fcn (with initial outputs)  N=[1]  D=[T_T_ST(7) 1]  Y0=MW0_ST(7)  U0=MW0_ST(7)
  出力制御遅れ有無 : Constant  Value=SW_T_ST(7)
  出力変化率 : RateLimiter  RisingSlewLimit=R_MWD_ST(7)/60  FallingSlewLimit=-R_MWD_ST(7)/60  SampleTimeMode=inherited  InitialCondition=MW0_ST(7)
  周波数バイアス : Lookup  InputValues=FX_FB_ST(:,7)/F0  Table=FY_FB_ST(:,7)  LookUpMeth=Interpolation-Use End Values
  圧力制御 : simulink_extras/Additional Linear/Transfer Fcn (with initial outputs)  N=[1]  D=[T3_B_ST(7) 1]  Y0=0  U0=0
  比例ゲイン : Gain  Gain=K_PREF_ST(7)
  積分時定数 : Gain  Gain=1/T_PREF_ST(7)
  蒸気加減弁開度 : Integrator  InitialCondition=MW0_ST(7)/PTH0_ST(7)  LimitOutput=on  UpperSaturationLimit=U_G_ST(7)  LowerSaturationLimit=L_G_ST(7)
  負荷 制限 : Switch  Threshold=0.5
  負荷 設定 : Switch  Threshold=0.5
  追従回路 : Subsystem
  速度調定率 : Gain  Gain=100/DELTA_ST(7)
  連続出力切替 : Subsystem
  運転モード : simulink/Logic and Bit Operations/Compare To Constant  relop=>=  const=L_MWD_ST(7)*GMW_ST(7)  OutDataTypeStr=boolean
  高圧タービン : simulink_extras/Additional Linear/Transfer Fcn (with initial outputs)  N=[1]  D=[T4_G_ST(7) 1]  Y0=MW0_ST(7)  U0=MW0_ST(7)
  高圧タービン分担比 : Gain  Gain=K_G_ST(7)
  タービン出力(MW) : Outport  VectorParamsAs1DForOutWhenUnconnected=off
  wires:
  運転モード/1 -> 連続出力切替/2(運転モード)
  LFC指令値(MW)/1 -> MWD(MW)/1
  EDC指令値(MW)/1 -> 運転モード/1, MWD(MW)/2
  出力制御遅れ有無/1 -> Switch3/2
  Switch3/1 -> 出力偏差/2
  出力制御遅れ/1 -> Switch3/1
  Switch1/1 -> Add/1
  Constant/1 -> Switch1/3
  周波数バイアス/1 -> Switch1/1
  負荷 制限/1 -> Ll/1, MinMax/1
  pu->MW/1 -> タービン出力(MW)/1
  連続出力切替/1(出力) -> pu->MW/1
  Hz->pu/1 -> 周波数バイアス/1, 速度調定率/1
  MW->pu/1 -> 連続出力切替/3(MWD), 出力変化率/1, MWD/1
  Switch2/1 -> Add2/2
  追従回路/1(Out) -> 負荷 設定/3, 負荷 制限/1
  負荷 設定/1 -> Pref/1, Subtract1/1
  GF運転・LL運転/1 -> Switch1/2, Switch2/2, 負荷 制限/2, 負荷 設定/2
  出力上下限/1 -> Switch3/3, 出力制御遅れ/1, MWDD/1, ボイラ発生蒸気/1
  Subtract/1 -> 圧力制御/1, ボイラ特性/1
  圧力制御/1 -> 主蒸気圧力 偏差/2
  ボイラ特性/1 -> 主蒸気圧力 偏差/1
  Add2/1 -> 追従回路/1(In)
  GF・LL幅/1 -> Add2/1
  タービン出力/1 -> 連続出力切替/1(モデル), PG_CURRENT(pu)/1, 出力偏差/1
  中低圧タービン分担比/1 -> タービン出力/1
  高圧タービン分担比/1 -> タービン出力/2
  中低圧タービン・再熱器/1 -> 中低圧タービン分担比/1
  高圧タービン/1 -> 高圧タービン分担比/1, 中低圧タービン・再熱器/1
  蒸気加減弁開度/1 -> Cv/1, Subtract2/2, 主蒸気流量/2
  CVサーボ開閉時間/1 -> 蒸気加減弁開度/1
  CVサーボ時定数/1 -> CVサーボ開閉時間/1
  Subtract2/1 -> CVサーボ時定数/1
  MinMax/1 -> Switch2/1, Subtract2/1
  スピードリレー/1 -> Subtract1/2
  主蒸気圧力/1 -> Pth/1, 主蒸気流量/1
  Subtract1/1 -> MinMax/2
  速度調定率/1 -> スピードリレー/1
  出力制御積分/1 -> Add3/2
  積分時定数/1 -> 出力制御積分/1
  主蒸気流量/1 -> 高圧タービン/1, Subtract/2
  主蒸気圧力設定/1 -> 主蒸気圧力/2, Pthd/1
  主蒸気圧力 偏差/1 -> 出力偏差/3, 主蒸気圧力/1
  Add3/1 -> 負荷 設定/1, Switch2/3, 負荷 制限/3
  比例ゲイン/1 -> Add3/1
  出力偏差/1 -> 積分時定数/1, 比例ゲイン/1
  ボイラ発生蒸気/1 -> 主蒸気圧力設定/1, Subtract/1
  出力変化率/1 -> Add/2
  Add/1 -> 出力上下限/1
  周波数偏差(Hz)/1 -> Hz->pu/1
  MWD(MW)/1 -> MW->pu/1

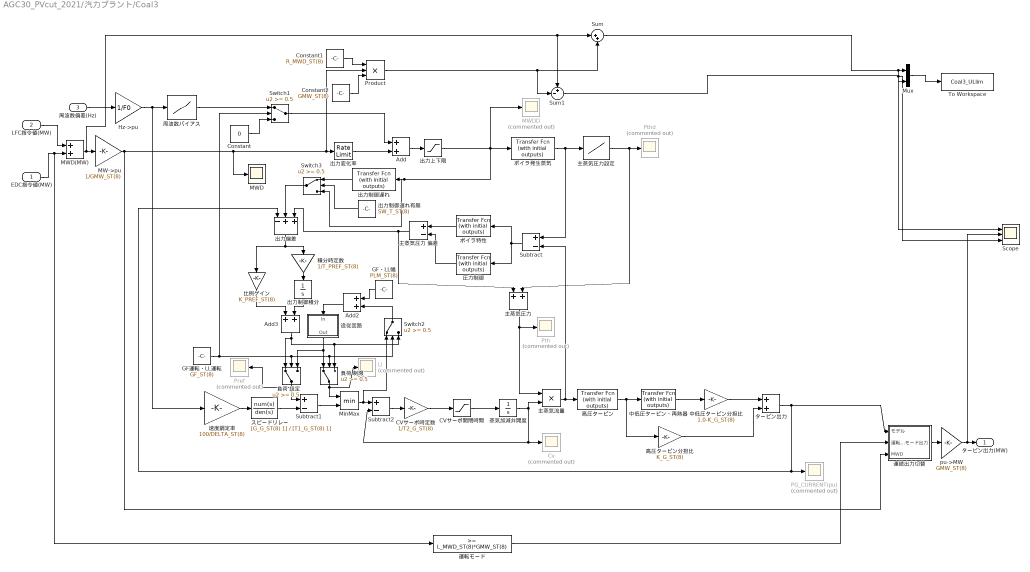
== system AGC30_PVcut_2021/汽力プラント/Coal3 ==
  EDC指令値(MW) : Inport
  LFC指令値(MW) : Inport  Port=2
  周波数偏差(Hz) : Inport  Port=3
  Add : Sum
  Add2 : Sum
  Add3 : Sum
  CVサーボ時定数 : Gain  Gain=1/T2_G_ST(8)
  CVサーボ開閉時間 : Saturate  UpperLimit=1/T3_G_ST(8)  LowerLimit=1/T6_G_ST(8)
  Constant : Constant  Value=0
  Constant1 : Constant  Value=R_MWD_ST(8)
  Constant2 : Constant  Value=GMW_ST(8)
  Cv : Scope  Commented=on
  GF・LL幅 : Constant  Value=PLM_ST(8)
  GF運転・LL運転 : Constant  Value=GF_ST(8)
  Hz->pu : Gain  Gain=1/F0
  Ll : Scope  Commented=on
  MW->pu : Gain  Gain=1/GMW_ST(8)
  MWD : Scope
  MWD(MW) : Sum
  MWDD : Scope  Commented=on
  MinMax : MinMax  Inputs=2
  Mux : Mux  Inputs=2
  PG_CURRENT(pu) : Scope  Commented=on
  Pref : Scope  Commented=on
  Product : Product  Inputs=3
  Pth : Scope  Commented=on
  Pthd : Scope  Commented=on
  Scope : Scope  NumInputPorts=3
  Subtract : Sum  Inputs=+-
  Subtract1 : Sum  Inputs=+-
  Subtract2 : Sum  Inputs=+-
  Sum : Sum  Inputs=|++
  Sum1 : Sum  Inputs=+-|
  Switch1 : Switch  Threshold=0.5
  Switch2 : Switch  Threshold=0.5
  Switch3 : Switch  Threshold=0.5
  To Workspace : ToWorkspace  VariableName=Coal3_ULlim  SampleTime=-1
      settings: Decimation=10  Save2DSignal=2-D array (concatenate along first dimension)
  pu->MW : Gain  Gain=GMW_ST(8)
  スピードリレー : TransferFcn  Numerator=[G_G_ST(8) 1]  Denominator=[T1_G_ST(8) 1]
  タービン出力 : Sum
  ボイラ特性 : simulink_extras/Additional Linear/Transfer Fcn (with initial outputs)  N=[1]  D=[T2_B_ST(8) 1]  Y0=0  U0=0
  ボイラ発生蒸気 : simulink_extras/Additional Linear/Transfer Fcn (with initial outputs)  N=[1]  D=[T1_B_ST(8) 1]  Y0=MW0_ST(8)  U0=MW0_ST(8)
  中低圧タービン・再熱器 : simulink_extras/Additional Linear/Transfer Fcn (with initial outputs)  N=[1]  D=[T5_G_ST(8) 1]  Y0=MW0_ST(8)  U0=MW0_ST(8)
  中低圧タービン分担比 : Gain  Gain=1.0-K_G_ST(8)
  主蒸気圧力 : Sum
  主蒸気圧力 偏差 : Sum  Inputs=+-
  主蒸気圧力設定 : Lookup  InputValues=FX_PTHD_ST(:,8)  Table=FY_PTHD_ST(:,8)  LookUpMeth=Interpolation-Use End Values
  主蒸気流量 : Product  RndMeth=Zero
  出力上下限 : Saturate  UpperLimit=U_MWD_ST(8)  LowerLimit=L_MWD_ST(8)
  出力偏差 : Sum  Inputs=-++
  出力制御積分 : Integrator  InitialCondition=MW0_ST(8)/PTH0_ST(8)  LimitOutput=on  UpperSaturationLimit=U_PREF_ST(8)  LowerSaturationLimit=L_PREF_ST(8)
  出力制御遅れ : simulink_extras/Additional Linear/Transfer Fcn (with initial outputs)  N=[1]  D=[T_T_ST(8) 1]  Y0=MW0_ST(8)  U0=MW0_ST(8)
  出力制御遅れ有無 : Constant  Value=SW_T_ST(8)
  出力変化率 : RateLimiter  RisingSlewLimit=R_MWD_ST(8)/60  FallingSlewLimit=-R_MWD_ST(8)/60  SampleTimeMode=inherited  InitialCondition=MW0_ST(8)
  周波数バイアス : Lookup  InputValues=FX_FB_ST(:,8)/F0  Table=FY_FB_ST(:,8)  LookUpMeth=Interpolation-Use End Values
  圧力制御 : simulink_extras/Additional Linear/Transfer Fcn (with initial outputs)  N=[1]  D=[T3_B_ST(8) 1]  Y0=0  U0=0
  比例ゲイン : Gain  Gain=K_PREF_ST(8)
  積分時定数 : Gain  Gain=1/T_PREF_ST(8)
  蒸気加減弁開度 : Integrator  InitialCondition=MW0_ST(8)/PTH0_ST(8)  LimitOutput=on  UpperSaturationLimit=U_G_ST(8)  LowerSaturationLimit=L_G_ST(8)
  負荷 制限 : Switch  Threshold=0.5
  負荷 設定 : Switch  Threshold=0.5
  追従回路 : Subsystem
  速度調定率 : Gain  Gain=100/DELTA_ST(8)
  連続出力切替 : Subsystem
  運転モード : simulink/Logic and Bit Operations/Compare To Constant  relop=>=  const=L_MWD_ST(8)*GMW_ST(8)  OutDataTypeStr=boolean
  高圧タービン : simulink_extras/Additional Linear/Transfer Fcn (with initial outputs)  N=[1]  D=[T4_G_ST(8) 1]  Y0=MW0_ST(8)  U0=MW0_ST(8)
  高圧タービン分担比 : Gain  Gain=K_G_ST(8)
  タービン出力(MW) : Outport  VectorParamsAs1DForOutWhenUnconnected=off
  wires:
  MWD(MW)/1 -> Sum/1, Sum1/1, MW->pu/1
  周波数偏差(Hz)/1 -> Hz->pu/1
  Add/1 -> 出力上下限/1
  出力変化率/1 -> Add/2
  ボイラ発生蒸気/1 -> Subtract/1, 主蒸気圧力設定/1
  出力偏差/1 -> 比例ゲイン/1, 積分時定数/1
  比例ゲイン/1 -> Add3/1
  Add3/1 -> 負荷 制限/3, Switch2/3, 負荷 設定/1
  主蒸気圧力 偏差/1 -> 主蒸気圧力/1, 出力偏差/3
  主蒸気圧力設定/1 -> Pthd/1, 主蒸気圧力/2
  主蒸気流量/1 -> Subtract/2, 高圧タービン/1
  積分時定数/1 -> 出力制御積分/1
  出力制御積分/1 -> Add3/2
  速度調定率/1 -> スピードリレー/1
  Subtract1/1 -> MinMax/2
  主蒸気圧力/1 -> 主蒸気流量/1, Pth/1
  スピードリレー/1 -> Subtract1/2
  MinMax/1 -> Subtract2/1, Switch2/1
  Subtract2/1 -> CVサーボ時定数/1
  CVサーボ時定数/1 -> CVサーボ開閉時間/1
  CVサーボ開閉時間/1 -> 蒸気加減弁開度/1
  蒸気加減弁開度/1 -> 主蒸気流量/2, Subtract2/2, Cv/1
  高圧タービン/1 -> 中低圧タービン・再熱器/1, 高圧タービン分担比/1
  中低圧タービン・再熱器/1 -> 中低圧タービン分担比/1
  高圧タービン分担比/1 -> タービン出力/2
  中低圧タービン分担比/1 -> タービン出力/1
  タービン出力/1 -> 出力偏差/1, PG_CURRENT(pu)/1, 連続出力切替/1(モデル)
  GF・LL幅/1 -> Add2/1
  Add2/1 -> 追従回路/1(In)
  ボイラ特性/1 -> 主蒸気圧力 偏差/1
  圧力制御/1 -> 主蒸気圧力 偏差/2
  Subtract/1 -> ボイラ特性/1, 圧力制御/1
  出力上下限/1 -> ボイラ発生蒸気/1, MWDD/1, Switch3/3, 出力制御遅れ/1
  GF運転・LL運転/1 -> 負荷 設定/2, 負荷 制限/2, Switch2/2, Switch1/2
  負荷 設定/1 -> Subtract1/1, Pref/1
  追従回路/1(Out) -> 負荷 制限/1, 負荷 設定/3
  Switch2/1 -> Add2/2
  MW->pu/1 -> MWD/1, Product/2, 出力変化率/1, 連続出力切替/3(MWD)
  Hz->pu/1 -> 速度調定率/1, 周波数バイアス/1
  連続出力切替/1(出力) -> pu->MW/1
  pu->MW/1 -> Scope/2, タービン出力(MW)/1
  負荷 制限/1 -> MinMax/1, Ll/1
  周波数バイアス/1 -> Switch1/1
  Constant/1 -> Switch1/3
  Switch1/1 -> Add/1
  出力制御遅れ/1 -> Switch3/1
  Switch3/1 -> 出力偏差/2
  出力制御遅れ有無/1 -> Switch3/2
  EDC指令値(MW)/1 -> MWD(MW)/2, 運転モード/1
  LFC指令値(MW)/1 -> MWD(MW)/1
  運転モード/1 -> 連続出力切替/2(運転モード)
  Constant1/1 -> Product/1
  Constant2/1 -> Product/3
  Product/1 -> Sum/2, Sum1/2
  Sum/1 -> Scope/1, Mux/1
  Sum1/1 -> Scope/3, Mux/2
  Mux/1 -> To Workspace/1

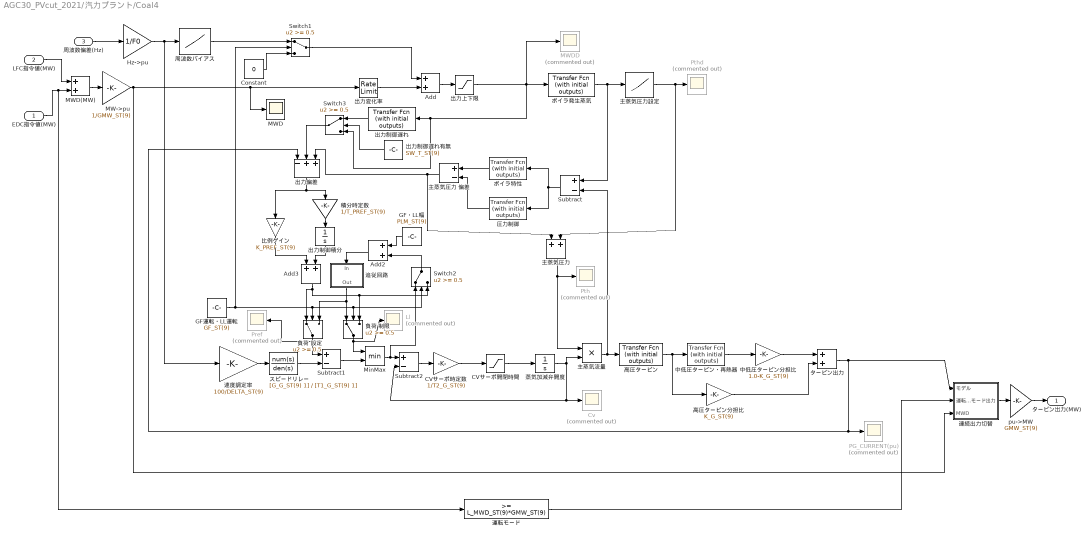
== system AGC30_PVcut_2021/汽力プラント/Coal4 ==
  EDC指令値(MW) : Inport
  LFC指令値(MW) : Inport  Port=2
  周波数偏差(Hz) : Inport  Port=3
  Add : Sum
  Add2 : Sum
  Add3 : Sum
  CVサーボ時定数 : Gain  Gain=1/T2_G_ST(9)
  CVサーボ開閉時間 : Saturate  UpperLimit=1/T3_G_ST(9)  LowerLimit=1/T6_G_ST(9)
  Constant : Constant  Value=0
  Cv : Scope  Commented=on
  GF・LL幅 : Constant  Value=PLM_ST(9)
  GF運転・LL運転 : Constant  Value=GF_ST(9)
  Hz->pu : Gain  Gain=1/F0
  Ll : Scope  Commented=on
  MW->pu : Gain  Gain=1/GMW_ST(9)
  MWD : Scope
  MWD(MW) : Sum
  MWDD : Scope  Commented=on
  MinMax : MinMax  Inputs=2
  PG_CURRENT(pu) : Scope  Commented=on
  Pref : Scope  Commented=on
  Pth : Scope  Commented=on
  Pthd : Scope  Commented=on
  Subtract : Sum  Inputs=+-
  Subtract1 : Sum  Inputs=+-
  Subtract2 : Sum  Inputs=+-
  Switch1 : Switch  Threshold=0.5
  Switch2 : Switch  Threshold=0.5
  Switch3 : Switch  Threshold=0.5
  pu->MW : Gain  Gain=GMW_ST(9)
  スピードリレー : TransferFcn  Numerator=[G_G_ST(9) 1]  Denominator=[T1_G_ST(9) 1]
  タービン出力 : Sum
  ボイラ特性 : simulink_extras/Additional Linear/Transfer Fcn (with initial outputs)  N=[1]  D=[T2_B_ST(9) 1]  Y0=0  U0=0
  ボイラ発生蒸気 : simulink_extras/Additional Linear/Transfer Fcn (with initial outputs)  N=[1]  D=[T1_B_ST(9) 1]  Y0=MW0_ST(9)  U0=MW0_ST(9)
  中低圧タービン・再熱器 : simulink_extras/Additional Linear/Transfer Fcn (with initial outputs)  N=[1]  D=[T5_G_ST(9) 1]  Y0=MW0_ST(9)  U0=MW0_ST(9)
  中低圧タービン分担比 : Gain  Gain=1.0-K_G_ST(9)
  主蒸気圧力 : Sum
  主蒸気圧力 偏差 : Sum  Inputs=+-
  主蒸気圧力設定 : Lookup  InputValues=FX_PTHD_ST(:,9)  Table=FY_PTHD_ST(:,9)  LookUpMeth=Interpolation-Use End Values
  主蒸気流量 : Product  RndMeth=Zero
  出力上下限 : Saturate  UpperLimit=U_MWD_ST(9)  LowerLimit=L_MWD_ST(9)
  出力偏差 : Sum  Inputs=-++
  出力制御積分 : Integrator  InitialCondition=MW0_ST(9)/PTH0_ST(9)  LimitOutput=on  UpperSaturationLimit=U_PREF_ST(9)  LowerSaturationLimit=L_PREF_ST(9)
  出力制御遅れ : simulink_extras/Additional Linear/Transfer Fcn (with initial outputs)  N=[1]  D=[T_T_ST(9) 1]  Y0=MW0_ST(9)  U0=MW0_ST(9)
  出力制御遅れ有無 : Constant  Value=SW_T_ST(9)
  出力変化率 : RateLimiter  RisingSlewLimit=R_MWD_ST(9)/60  FallingSlewLimit=-R_MWD_ST(9)/60  SampleTimeMode=inherited  InitialCondition=MW0_ST(9)
  周波数バイアス : Lookup  InputValues=FX_FB_ST(:,9)/F0  Table=FY_FB_ST(:,9)  LookUpMeth=Interpolation-Use End Values
  圧力制御 : simulink_extras/Additional Linear/Transfer Fcn (with initial outputs)  N=[1]  D=[T3_B_ST(9) 1]  Y0=0  U0=0
  比例ゲイン : Gain  Gain=K_PREF_ST(9)
  積分時定数 : Gain  Gain=1/T_PREF_ST(9)
  蒸気加減弁開度 : Integrator  InitialCondition=MW0_ST(9)/PTH0_ST(9)  LimitOutput=on  UpperSaturationLimit=U_G_ST(9)  LowerSaturationLimit=L_G_ST(9)
  負荷 制限 : Switch  Threshold=0.5
  負荷 設定 : Switch  Threshold=0.5
  追従回路 : Subsystem
  速度調定率 : Gain  Gain=100/DELTA_ST(9)
  連続出力切替 : Subsystem
  運転モード : simulink/Logic and Bit Operations/Compare To Constant  relop=>=  const=L_MWD_ST(9)*GMW_ST(9)  OutDataTypeStr=boolean
  高圧タービン : simulink_extras/Additional Linear/Transfer Fcn (with initial outputs)  N=[1]  D=[T4_G_ST(9) 1]  Y0=MW0_ST(9)  U0=MW0_ST(9)
  高圧タービン分担比 : Gain  Gain=K_G_ST(9)
  タービン出力(MW) : Outport  VectorParamsAs1DForOutWhenUnconnected=off
  wires:
  MWD(MW)/1 -> MW->pu/1
  周波数偏差(Hz)/1 -> Hz->pu/1
  Add/1 -> 出力上下限/1
  出力変化率/1 -> Add/2
  ボイラ発生蒸気/1 -> Subtract/1, 主蒸気圧力設定/1
  出力偏差/1 -> 比例ゲイン/1, 積分時定数/1
  比例ゲイン/1 -> Add3/1
  Add3/1 -> 負荷 制限/3, Switch2/3, 負荷 設定/1
  主蒸気圧力 偏差/1 -> 主蒸気圧力/1, 出力偏差/3
  主蒸気圧力設定/1 -> Pthd/1, 主蒸気圧力/2
  主蒸気流量/1 -> Subtract/2, 高圧タービン/1
  積分時定数/1 -> 出力制御積分/1
  出力制御積分/1 -> Add3/2
  速度調定率/1 -> スピードリレー/1
  Subtract1/1 -> MinMax/2
  主蒸気圧力/1 -> 主蒸気流量/1, Pth/1
  スピードリレー/1 -> Subtract1/2
  MinMax/1 -> Subtract2/1, Switch2/1
  Subtract2/1 -> CVサーボ時定数/1
  CVサーボ時定数/1 -> CVサーボ開閉時間/1
  CVサーボ開閉時間/1 -> 蒸気加減弁開度/1
  蒸気加減弁開度/1 -> 主蒸気流量/2, Subtract2/2, Cv/1
  高圧タービン/1 -> 中低圧タービン・再熱器/1, 高圧タービン分担比/1
  中低圧タービン・再熱器/1 -> 中低圧タービン分担比/1
  高圧タービン分担比/1 -> タービン出力/2
  中低圧タービン分担比/1 -> タービン出力/1
  タービン出力/1 -> 出力偏差/1, PG_CURRENT(pu)/1, 連続出力切替/1(モデル)
  GF・LL幅/1 -> Add2/1
  Add2/1 -> 追従回路/1(In)
  ボイラ特性/1 -> 主蒸気圧力 偏差/1
  圧力制御/1 -> 主蒸気圧力 偏差/2
  Subtract/1 -> ボイラ特性/1, 圧力制御/1
  出力上下限/1 -> ボイラ発生蒸気/1, MWDD/1, 出力制御遅れ/1, Switch3/3
  GF運転・LL運転/1 -> 負荷 設定/2, 負荷 制限/2, Switch2/2, Switch1/2
  負荷 設定/1 -> Subtract1/1, Pref/1
  追従回路/1(Out) -> 負荷 制限/1, 負荷 設定/3
  Switch2/1 -> Add2/2
  MW->pu/1 -> MWD/1, 出力変化率/1, 連続出力切替/3(MWD)
  Hz->pu/1 -> 速度調定率/1, 周波数バイアス/1
  連続出力切替/1(出力) -> pu->MW/1
  pu->MW/1 -> タービン出力(MW)/1
  負荷 制限/1 -> MinMax/1, Ll/1
  周波数バイアス/1 -> Switch1/1
  Constant/1 -> Switch1/3
  Switch1/1 -> Add/1
  出力制御遅れ/1 -> Switch3/1
  Switch3/1 -> 出力偏差/2
  出力制御遅れ有無/1 -> Switch3/2
  EDC指令値(MW)/1 -> MWD(MW)/2, 運転モード/1
  LFC指令値(MW)/1 -> MWD(MW)/1
  運転モード/1 -> 連続出力切替/2(運転モード)

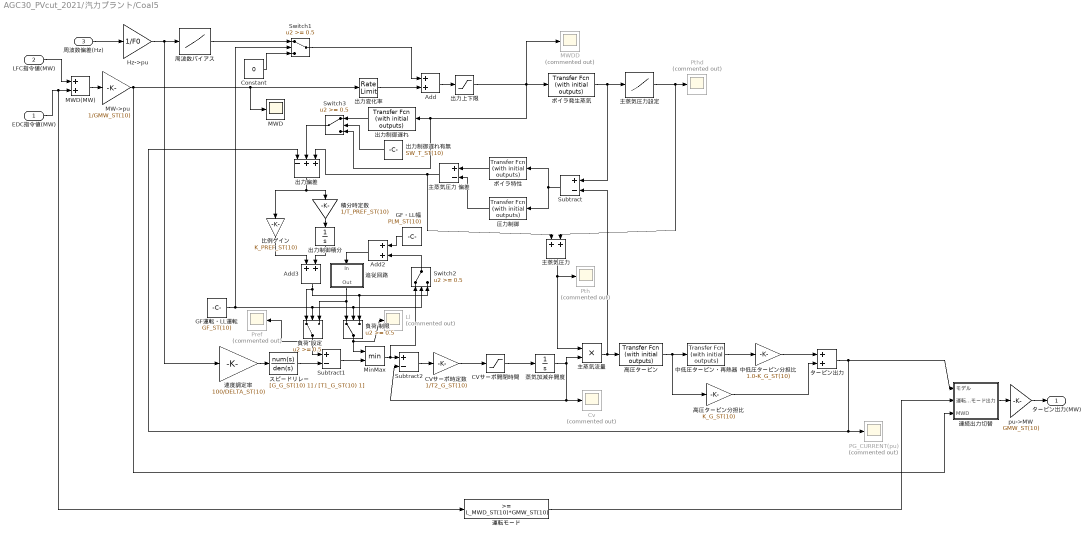
== system AGC30_PVcut_2021/汽力プラント/Coal5 ==
  EDC指令値(MW) : Inport
  LFC指令値(MW) : Inport  Port=2
  周波数偏差(Hz) : Inport  Port=3
  Add : Sum
  Add2 : Sum
  Add3 : Sum
  CVサーボ時定数 : Gain  Gain=1/T2_G_ST(10)
  CVサーボ開閉時間 : Saturate  UpperLimit=1/T3_G_ST(10)  LowerLimit=1/T6_G_ST(10)
  Constant : Constant  Value=0
  Cv : Scope  Commented=on
  GF・LL幅 : Constant  Value=PLM_ST(10)
  GF運転・LL運転 : Constant  Value=GF_ST(10)
  Hz->pu : Gain  Gain=1/F0
  Ll : Scope  Commented=on
  MW->pu : Gain  Gain=1/GMW_ST(10)
  MWD : Scope
  MWD(MW) : Sum
  MWDD : Scope  Commented=on
  MinMax : MinMax  Inputs=2
  PG_CURRENT(pu) : Scope  Commented=on
  Pref : Scope  Commented=on
  Pth : Scope  Commented=on
  Pthd : Scope  Commented=on
  Subtract : Sum  Inputs=+-
  Subtract1 : Sum  Inputs=+-
  Subtract2 : Sum  Inputs=+-
  Switch1 : Switch  Threshold=0.5
  Switch2 : Switch  Threshold=0.5
  Switch3 : Switch  Threshold=0.5
  pu->MW : Gain  Gain=GMW_ST(10)
  スピードリレー : TransferFcn  Numerator=[G_G_ST(10) 1]  Denominator=[T1_G_ST(10) 1]
  タービン出力 : Sum
  ボイラ特性 : simulink_extras/Additional Linear/Transfer Fcn (with initial outputs)  N=[1]  D=[T2_B_ST(10) 1]  Y0=0  U0=0
  ボイラ発生蒸気 : simulink_extras/Additional Linear/Transfer Fcn (with initial outputs)  N=[1]  D=[T1_B_ST(10) 1]  Y0=MW0_ST(10)  U0=MW0_ST(10)
  中低圧タービン・再熱器 : simulink_extras/Additional Linear/Transfer Fcn (with initial outputs)  N=[1]  D=[T5_G_ST(10) 1]  Y0=MW0_ST(10)  U0=MW0_ST(10)
  中低圧タービン分担比 : Gain  Gain=1.0-K_G_ST(10)
  主蒸気圧力 : Sum
  主蒸気圧力 偏差 : Sum  Inputs=+-
  主蒸気圧力設定 : Lookup  InputValues=FX_PTHD_ST(:,10)  Table=FY_PTHD_ST(:,10)  LookUpMeth=Interpolation-Use End Values
  主蒸気流量 : Product  RndMeth=Zero
  出力上下限 : Saturate  UpperLimit=U_MWD_ST(10)  LowerLimit=L_MWD_ST(10)
  出力偏差 : Sum  Inputs=-++
  出力制御積分 : Integrator  InitialCondition=MW0_ST(10)/PTH0_ST(10)  LimitOutput=on  UpperSaturationLimit=U_PREF_ST(10)  LowerSaturationLimit=L_PREF_ST(10)
  出力制御遅れ : simulink_extras/Additional Linear/Transfer Fcn (with initial outputs)  N=[1]  D=[T_T_ST(10) 1]  Y0=MW0_ST(10)  U0=MW0_ST(10)
  出力制御遅れ有無 : Constant  Value=SW_T_ST(10)
  出力変化率 : RateLimiter  RisingSlewLimit=R_MWD_ST(10)/60  FallingSlewLimit=-R_MWD_ST(10)/60  SampleTimeMode=inherited  InitialCondition=MW0_ST(10)
  周波数バイアス : Lookup  InputValues=FX_FB_ST(:,10)/F0  Table=FY_FB_ST(:,10)  LookUpMeth=Interpolation-Use End Values
  圧力制御 : simulink_extras/Additional Linear/Transfer Fcn (with initial outputs)  N=[1]  D=[T3_B_ST(10) 1]  Y0=0  U0=0
  比例ゲイン : Gain  Gain=K_PREF_ST(10)
  積分時定数 : Gain  Gain=1/T_PREF_ST(10)
  蒸気加減弁開度 : Integrator  InitialCondition=MW0_ST(10)/PTH0_ST(10)  LimitOutput=on  UpperSaturationLimit=U_G_ST(10)  LowerSaturationLimit=L_G_ST(10)
  負荷 制限 : Switch  Threshold=0.5
  負荷 設定 : Switch  Threshold=0.5
  追従回路 : Subsystem
  速度調定率 : Gain  Gain=100/DELTA_ST(10)
  連続出力切替 : Subsystem
  運転モード : simulink/Logic and Bit Operations/Compare To Constant  relop=>=  const=L_MWD_ST(10)*GMW_ST(10)  OutDataTypeStr=boolean
  高圧タービン : simulink_extras/Additional Linear/Transfer Fcn (with initial outputs)  N=[1]  D=[T4_G_ST(10) 1]  Y0=MW0_ST(10)  U0=MW0_ST(10)
  高圧タービン分担比 : Gain  Gain=K_G_ST(10)
  タービン出力(MW) : Outport  VectorParamsAs1DForOutWhenUnconnected=off
  wires:
  MWD(MW)/1 -> MW->pu/1
  周波数偏差(Hz)/1 -> Hz->pu/1
  Add/1 -> 出力上下限/1
  出力変化率/1 -> Add/2
  ボイラ発生蒸気/1 -> Subtract/1, 主蒸気圧力設定/1
  出力偏差/1 -> 比例ゲイン/1, 積分時定数/1
  比例ゲイン/1 -> Add3/1
  Add3/1 -> 負荷 制限/3, Switch2/3, 負荷 設定/1
  主蒸気圧力 偏差/1 -> 主蒸気圧力/1, 出力偏差/3
  主蒸気圧力設定/1 -> Pthd/1, 主蒸気圧力/2
  主蒸気流量/1 -> Subtract/2, 高圧タービン/1
  積分時定数/1 -> 出力制御積分/1
  出力制御積分/1 -> Add3/2
  速度調定率/1 -> スピードリレー/1
  Subtract1/1 -> MinMax/2
  主蒸気圧力/1 -> 主蒸気流量/1, Pth/1
  スピードリレー/1 -> Subtract1/2
  MinMax/1 -> Subtract2/1, Switch2/1
  Subtract2/1 -> CVサーボ時定数/1
  CVサーボ時定数/1 -> CVサーボ開閉時間/1
  CVサーボ開閉時間/1 -> 蒸気加減弁開度/1
  蒸気加減弁開度/1 -> 主蒸気流量/2, Subtract2/2, Cv/1
  高圧タービン/1 -> 中低圧タービン・再熱器/1, 高圧タービン分担比/1
  中低圧タービン・再熱器/1 -> 中低圧タービン分担比/1
  高圧タービン分担比/1 -> タービン出力/2
  中低圧タービン分担比/1 -> タービン出力/1
  タービン出力/1 -> 出力偏差/1, PG_CURRENT(pu)/1, 連続出力切替/1(モデル)
  GF・LL幅/1 -> Add2/1
  Add2/1 -> 追従回路/1(In)
  ボイラ特性/1 -> 主蒸気圧力 偏差/1
  圧力制御/1 -> 主蒸気圧力 偏差/2
  Subtract/1 -> ボイラ特性/1, 圧力制御/1
  出力上下限/1 -> ボイラ発生蒸気/1, MWDD/1, 出力制御遅れ/1, Switch3/3
  GF運転・LL運転/1 -> 負荷 設定/2, 負荷 制限/2, Switch2/2, Switch1/2
  負荷 設定/1 -> Subtract1/1, Pref/1
  追従回路/1(Out) -> 負荷 制限/1, 負荷 設定/3
  Switch2/1 -> Add2/2
  MW->pu/1 -> MWD/1, 出力変化率/1, 連続出力切替/3(MWD)
  Hz->pu/1 -> 速度調定率/1, 周波数バイアス/1
  連続出力切替/1(出力) -> pu->MW/1
  pu->MW/1 -> タービン出力(MW)/1
  負荷 制限/1 -> MinMax/1, Ll/1
  周波数バイアス/1 -> Switch1/1
  Constant/1 -> Switch1/3
  Switch1/1 -> Add/1
  出力制御遅れ/1 -> Switch3/1
  Switch3/1 -> 出力偏差/2
  出力制御遅れ有無/1 -> Switch3/2
  EDC指令値(MW)/1 -> MWD(MW)/2, 運転モード/1
  LFC指令値(MW)/1 -> MWD(MW)/1
  運転モード/1 -> 連続出力切替/2(運転モード)
